simulink model "IMU_with_set_pace"  (R2024a)
settings: Solver=VariableStepAuto  StartTime=0.0  StopTime=10.0  RelTol=1e-3
libraries: MecRoKa_SFunction_Library x3, aerolibanimutils x1
settings Model: Creator=saura  LastModifiedBy=Ishant
settings RTWCC: GPUComputeCapability=3.5

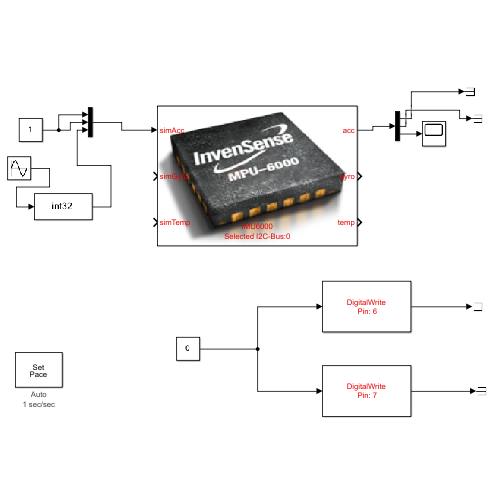
[thumbnail: Simulink's stored preview of the top-level diagram]
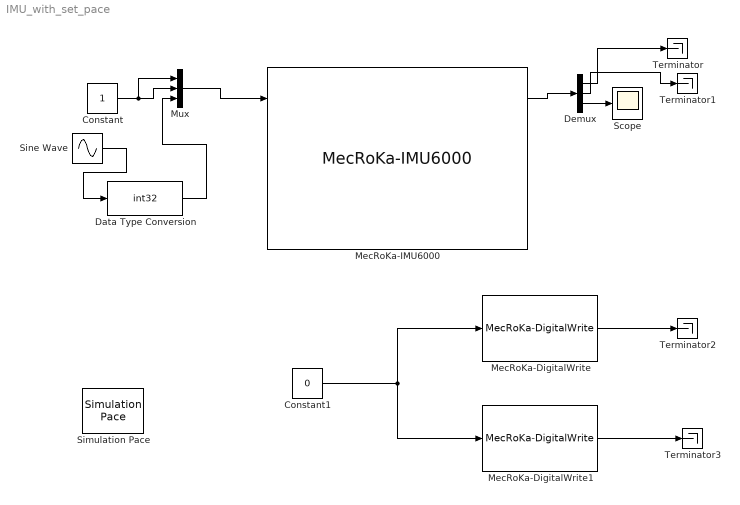
== system IMU_with_set_pace ==
  Constant : Constant  OutDataTypeStr=int32
  Constant1 : Constant  Value=0  OutDataTypeStr=boolean
  Data Type Conversion : DataTypeConversion  OutDataTypeStr=int32  SaturateOnIntegerOverflow=off  RndMeth=Floor
  Demux : Demux  Outputs=3
  MecRoKa-DigitalWrite : MecRoKa_SFunction_Library/Arduino-Blocks/Arduino-Library/MecRoKa-DigitalWrite  pinNumber=6
      settings: SourceProductName=MecRoKa_SFunction-Library
  MecRoKa-DigitalWrite1 : MecRoKa_SFunction_Library/Arduino-Blocks/Arduino-Library/MecRoKa-DigitalWrite  pinNumber=7
      settings: SourceProductName=MecRoKa_SFunction-Library
  MecRoKa-IMU6000 : MecRoKa_SFunction_Library/Arduino-Blocks/Sensor-Library/MecRoKa-IMU6000  selectWire=0
      settings: SourceProductName=MecRoKa_SFunction-Library
  Mux : Mux  Inputs=3
  Scope : Scope
  Simulation Pace : aerolibanimutils/Simulation Pace  SimulationPace=1  SleepMode=Auto  OutputPaceError=off  SampleTime=1/30
  Sine Wave : Sin  SampleTime=0
  Terminator{,1..3} (4 alike) : Terminator
  wires:
  Constant/1 -> Mux/1, Mux/2
  Mux/1 -> MecRoKa-IMU6000/1
  Demux/3 -> Scope/1
  MecRoKa-IMU6000/1 -> Demux/1
  Demux/1 -> Terminator/1
  Demux/2 -> Terminator1/1
  Sine Wave/1 -> Data Type Conversion/1
  Data Type Conversion/1 -> Mux/3
  Constant1/1 -> MecRoKa-DigitalWrite/1, MecRoKa-DigitalWrite1/1
  MecRoKa-DigitalWrite/1 -> Terminator2/1
  MecRoKa-DigitalWrite1/1 -> Terminator3/1
